simulink model "visualize_r2018a"  (R2018a)
settings: Solver=VariableStepAuto  StartTime=0.0  StopTime=inf  RelTol=1e-3
PostLoadFcn:
  | b = [0 0 0];
  | A = eye(3);
undefined symbols (not defined in the file or in its folder): NULL, serial
libraries: instrumentlib x2
settings Model: OrderedModelArguments=off  Creator=alvin  LastModifiedBy=alvin
settings DataIOCC: ReturnWorkspaceOutputs=on
settings SFSimCC: SimUseLocalCustomCode=on
settings RTWCC: RTWUseLocalCustomCode=on

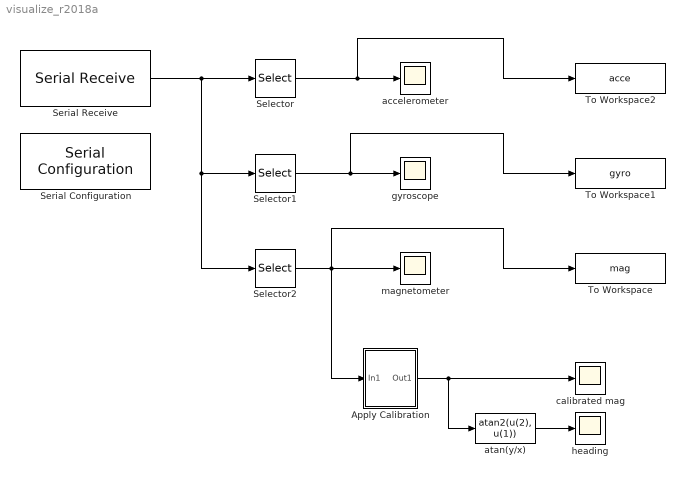
== system visualize_r2018a ==
  Apply Calibration : Subsystem
  Selector : Selector  NumberOfDimensions=2  InputPortWidth=3  IndexOptions=Select all,Index vector (dialog)  Indices=[1 3],1  OutputSizes=1,1
  Selector1 : Selector  NumberOfDimensions=2  InputPortWidth=3  IndexOptions=Select all,Index vector (dialog)  Indices=[1 3],2  OutputSizes=1,1
  Selector2 : Selector  NumberOfDimensions=2  InputPortWidth=3  IndexOptions=Select all,Index vector (dialog)  Indices=[1 3],3  OutputSizes=1,1
  Serial Configuration : instrumentlib/Serial Configuration  Priority=-200000  ComPortMenu=<Please select a port...>  ComPort=/dev/ttyACM0  ObjConstructor=serial('/dev/ttyACM0');  BaudRate=115200  DataBits=8  Parity=none  StopBits=1  FlowControl=none  Timeout=10  ByteOrder=LittleEndian
  Serial Receive : instrumentlib/Serial Receive  ComPortMenu=<Please select a port...>  ComPort=/dev/ttyACM0  ObjConstructor=serial('/dev/ttyACM0');  Header=s  Terminator=NULL ('\0')  DataSize="[3  3]"  DataType=single  EnableBlockingMode=on  ActionDataUnavailable=Output last received value  CustomValue=0  SampleTime=0.01
  To Workspace : ToWorkspace  VariableName=mag  SampleTime=-1
  To Workspace1 : ToWorkspace  VariableName=gyro  SampleTime=-1
  To Workspace2 : ToWorkspace  VariableName=acce  SampleTime=-1
  accelerometer : Scope
  atan(y/x) : Fcn  Expr=atan2(u(2), u(1))
  calibrated mag : Scope
  gyroscope : Scope
  heading : Scope
  magnetometer : Scope
  wires:
  Selector/1 -> To Workspace2/1, accelerometer/1
  Selector1/1 -> To Workspace1/1, gyroscope/1
  Selector2/1 -> Apply Calibration/1(In1), To Workspace/1, magnetometer/1
  Serial Receive/1 -> Selector1/1, Selector2/1, Selector/1
  atan(y/x)/1 -> heading/1
  Apply Calibration/1(Out1) -> atan(y/x)/1, calibrated mag/1

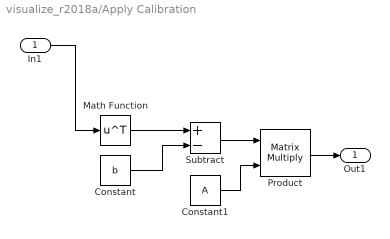
== system visualize_r2018a/Apply Calibration ==
  In1 : Inport
  Constant : Constant  Value=b  VectorParams1D=off
  Constant1 : Constant  Value=A  VectorParams1D=off
  Math Function : Math  Operator=transpose  SaturateOnIntegerOverflow=on
  Product : Product  Multiplication=Matrix(*)
  Subtract : Sum  Inputs=+-
  Out1 : Outport
  wires:
  Constant/1 -> Subtract/2
  Math Function/1 -> Subtract/1
  In1/1 -> Math Function/1
  Product/1 -> Out1/1
  Subtract/1 -> Product/1
  Constant1/1 -> Product/2
